simulink model "FDMATest"  (R2024b)
settings: Solver=VariableStepAuto  StartTime=0.0  StopTime=10.0  RelTol=1e-3
libraries: dspsrcs4 x12, dspfdesign x8

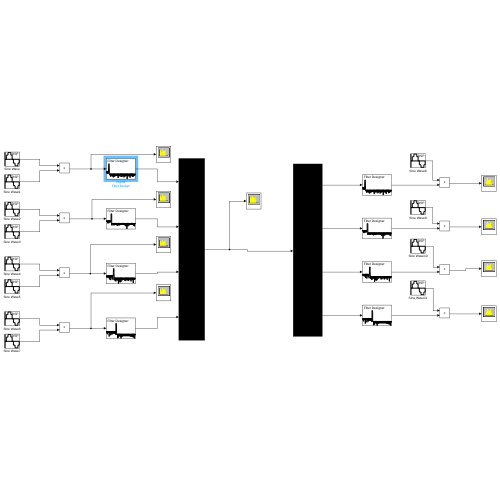
[thumbnail: Simulink's stored preview of the top-level diagram]
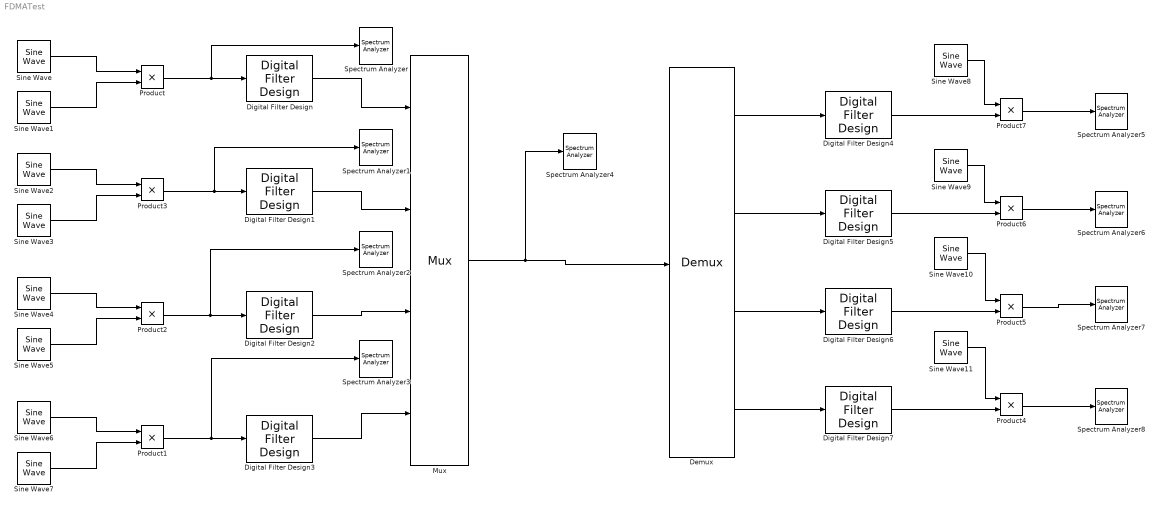
== system FDMATest ==
  Demux : Demux
  Digital Filter Design{,1..7} (8 alike) : dspfdesign/Digital Filter Design  mwdsp_browser_bugfix_var=off
  Mux : Mux
  Product{,1..7} (8 alike) : Product
  Sine Wave{,2,4,6} (4 alike) : dspsrcs4/Sine Wave  Amplitude=1  Frequency=20  Phase=0  SampleMode=Discrete  OutComplex=Real  CompMethod=Trigonometric fcn  TableSize=Speed  SampleTime=1/1000  SamplesPerFrame=1  ResetState=Restart at time zero  OutputFrames=off  dataType=double  wordLen=16  udDataType=sfix(16)  fracBitsMode=Best precision  numFracBits=15  OutDataTypeStr=double  LastOutDataTypeStr=double
  Sine Wave1 : dspsrcs4/Sine Wave  Amplitude=1  Frequency=100  Phase=0  SampleMode=Discrete  OutComplex=Real  CompMethod=Trigonometric fcn  TableSize=Speed  SampleTime=1/1000  SamplesPerFrame=1  ResetState=Restart at time zero  OutputFrames=off  dataType=double  wordLen=16  udDataType=sfix(16)  fracBitsMode=Best precision  numFracBits=15  OutDataTypeStr=double  LastOutDataTypeStr=double
  Sine Wave10 : dspsrcs4/Sine Wave  Amplitude=1  Frequency=300  Phase=0  SampleMode=Discrete  OutComplex=Real  CompMethod=Trigonometric fcn  TableSize=Speed  SampleTime=1/1000  SamplesPerFrame=1  ResetState=Restart at time zero  OutputFrames=off  dataType=double  wordLen=16  udDataType=sfix(16)  fracBitsMode=Best precision  numFracBits=15  OutDataTypeStr=double  LastOutDataTypeStr=double
  Sine Wave11 : dspsrcs4/Sine Wave  Amplitude=1  Frequency=400  Phase=0  SampleMode=Discrete  OutComplex=Real  CompMethod=Trigonometric fcn  TableSize=Speed  SampleTime=1/1000  SamplesPerFrame=1  ResetState=Restart at time zero  OutputFrames=off  dataType=double  wordLen=16  udDataType=sfix(16)  fracBitsMode=Best precision  numFracBits=15  OutDataTypeStr=double  LastOutDataTypeStr=double
  Sine Wave3 : dspsrcs4/Sine Wave  Amplitude=1  Frequency=200  Phase=0  SampleMode=Discrete  OutComplex=Real  CompMethod=Trigonometric fcn  TableSize=Speed  SampleTime=1/1000  SamplesPerFrame=1  ResetState=Restart at time zero  OutputFrames=off  dataType=double  wordLen=16  udDataType=sfix(16)  fracBitsMode=Best precision  numFracBits=15  OutDataTypeStr=double  LastOutDataTypeStr=double
  Sine Wave5 : dspsrcs4/Sine Wave  Amplitude=1  Frequency=300  Phase=0  SampleMode=Discrete  OutComplex=Real  CompMethod=Trigonometric fcn  TableSize=Speed  SampleTime=1/1000  SamplesPerFrame=1  ResetState=Restart at time zero  OutputFrames=off  dataType=double  wordLen=16  udDataType=sfix(16)  fracBitsMode=Best precision  numFracBits=15  OutDataTypeStr=double  LastOutDataTypeStr=double
  Sine Wave7 : dspsrcs4/Sine Wave  Amplitude=1  Frequency=400  Phase=0  SampleMode=Discrete  OutComplex=Real  CompMethod=Trigonometric fcn  TableSize=Speed  SampleTime=1/1000  SamplesPerFrame=1  ResetState=Restart at time zero  OutputFrames=off  dataType=double  wordLen=16  udDataType=sfix(16)  fracBitsMode=Best precision  numFracBits=15  OutDataTypeStr=double  LastOutDataTypeStr=double
  Sine Wave8 : dspsrcs4/Sine Wave  Amplitude=1  Frequency=100  Phase=0  SampleMode=Discrete  OutComplex=Real  CompMethod=Trigonometric fcn  TableSize=Speed  SampleTime=1/1000  SamplesPerFrame=1  ResetState=Restart at time zero  OutputFrames=off  dataType=double  wordLen=16  udDataType=sfix(16)  fracBitsMode=Best precision  numFracBits=15  OutDataTypeStr=double  LastOutDataTypeStr=double
  Sine Wave9 : dspsrcs4/Sine Wave  Amplitude=1  Frequency=200  Phase=0  SampleMode=Discrete  OutComplex=Real  CompMethod=Trigonometric fcn  TableSize=Speed  SampleTime=1/1000  SamplesPerFrame=1  ResetState=Restart at time zero  OutputFrames=off  dataType=double  wordLen=16  udDataType=sfix(16)  fracBitsMode=Best precision  numFracBits=15  OutDataTypeStr=double  LastOutDataTypeStr=double
  Spectrum Analyzer : SpectrumAnalyzer  WindowPosition=[1520.000000,830.000000,800.000000,500.000000,]  Visible=on  ScopeFrameLocation=window  WindowInvariantSamplesPerUpdate=on  YLimits=[-55.01079838,25.9672874]
  Spectrum Analyzer1 : SpectrumAnalyzer  WindowPosition=[853.400024,153.000000,342.000000,500.000000,]  Visible=on  ScopeFrameLocation=window  WindowInvariantSamplesPerUpdate=on  YLimits=[-42.63503311,23.41915527]
  Spectrum Analyzer2 : SpectrumAnalyzer  WindowPosition=[357.399994,641.599998,302.000000,2.400002,]  Visible=on  ScopeFrameLocation=window  WindowInvariantSamplesPerUpdate=on  YLimits=[-42.63503311,23.41915527]
  Spectrum Analyzer3 : SpectrumAnalyzer  WindowPosition=[20.400000,145.000000,342.000000,500.000000,]  Visible=on  ScopeFrameLocation=window  WindowInvariantSamplesPerUpdate=on  YLimits=[-55.01079838,25.9672874]
  Spectrum Analyzer4 : SpectrumAnalyzer  WindowPosition=[1520.000000,830.000000,800.000000,500.000000,]  Visible=on  ScopeFrameLocation=window  WindowInvariantSamplesPerUpdate=on  YLimits=[-121.17134569,-55.78607626]
  Spectrum Analyzer5 : SpectrumAnalyzer  WindowPosition=[1520.000000,830.000000,800.000000,500.000000,]  Visible=on  ScopeFrameLocation=window  WindowInvariantSamplesPerUpdate=on  YLimits=[-134.83206371,-43.38875602]
  Spectrum Analyzer6 : SpectrumAnalyzer  WindowPosition=[853.400024,153.000000,342.000000,500.000000,]  Visible=on  ScopeFrameLocation=window  WindowInvariantSamplesPerUpdate=on  YLimits=[-147.46645226,-57.06147369]
  Spectrum Analyzer7 : SpectrumAnalyzer  WindowPosition=[357.399994,641.599998,302.000000,2.400002,]  Visible=on  ScopeFrameLocation=window  WindowInvariantSamplesPerUpdate=on  YLimits=[-143.83426287,-66.10232782]
  Spectrum Analyzer8 : SpectrumAnalyzer  WindowPosition=[20.000000,145.000000,742.000000,500.000000,]  Visible=on  ScopeFrameLocation=window  WindowInvariantSamplesPerUpdate=on  YLimits=[-143.99125552,-73.69752245]
  wires:
  Sine Wave/1 -> Product/1
  Sine Wave1/1 -> Product/2
  Sine Wave2/1 -> Product3/1
  Sine Wave3/1 -> Product3/2
  Sine Wave4/1 -> Product2/1
  Sine Wave5/1 -> Product2/2
  Sine Wave6/1 -> Product1/1
  Sine Wave7/1 -> Product1/2
  Product/1 -> Spectrum Analyzer/1, Digital Filter Design/1
  Product3/1 -> Spectrum Analyzer1/1, Digital Filter Design1/1
  Product2/1 -> Spectrum Analyzer2/1, Digital Filter Design2/1
  Product1/1 -> Spectrum Analyzer3/1, Digital Filter Design3/1
  Digital Filter Design/1 -> Mux/1
  Digital Filter Design1/1 -> Mux/2
  Digital Filter Design2/1 -> Mux/3
  Digital Filter Design3/1 -> Mux/4
  Mux/1 -> Demux/1, Spectrum Analyzer4/1
  Product4/1 -> Spectrum Analyzer8/1
  Product5/1 -> Spectrum Analyzer7/1
  Product6/1 -> Spectrum Analyzer6/1
  Product7/1 -> Spectrum Analyzer5/1
  Sine Wave8/1 -> Product7/1
  Sine Wave9/1 -> Product6/1
  Sine Wave10/1 -> Product5/1
  Sine Wave11/1 -> Product4/1
  Digital Filter Design4/1 -> Product7/2
  Digital Filter Design5/1 -> Product6/2
  Digital Filter Design6/1 -> Product5/2
  Digital Filter Design7/1 -> Product4/2
  Demux/1 -> Digital Filter Design4/1
  Demux/2 -> Digital Filter Design5/1
  Demux/3 -> Digital Filter Design6/1
  Demux/4 -> Digital Filter Design7/1
